simulink model "sphero_ver_01"  (R2020b)
settings: Solver=VariableStepAuto  StartTime=0.0  StopTime=10.0  RelTol=1e-3
libraries: pid_lib x1
settings Model: Creator=filip  LastModifiedBy=filip

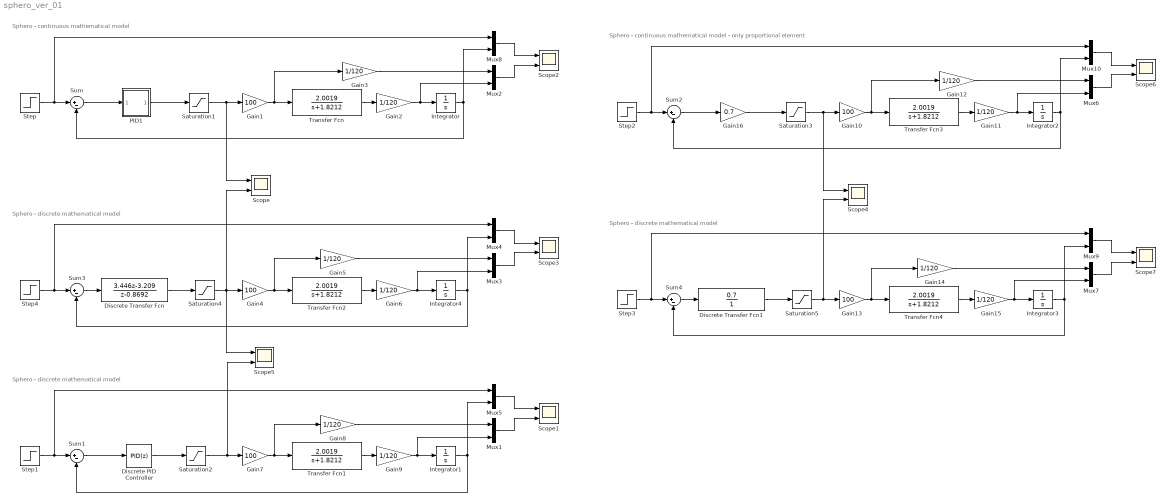
== system sphero_ver_01 ==
  note: Sphero - discrete mathematical model
  note: Sphero - continuous mathematical model
  note: Sphero - discrete mathematical model
  note: Sphero - continuous mathematical model - only proportional element
  note: Sphero - discrete mathematical model
  Discrete Transfer Fcn : DiscreteTransferFcn  Numerator=[3.446 -3.209]  Denominator=[1 -0.8692]  SampleTime=0.04
  Discrete Transfer Fcn1 : DiscreteTransferFcn  Numerator=[0.7]  Denominator=[1]  SampleTime=0.04
  Discrete PID Controller : pid_lib/PID Controller  Controller=PID  Form=Parallel  TimeDomain=Discrete-time  UseExternalTs=off  SampleTime=0.04  IntegratorMethod=Forward Euler  FilterMethod=Forward Euler  ControllerParametersSource=internal  P=1.81  I=0  D=0.5  UseFilter=on  N=3.5  TunerSelectOption=Transfer Function Based (PID Tuner App)  InitialConditionSource=internal  InitialConditionForIntegrator=0  InitialConditionForFilter=0  DifferentiatorICPrevScaledInput=0  ExternalReset=none  TrackingMode=off  Kt=1  LimitOutput=off  SatLimitsSource=internal  UpperSaturationLimit=inf  LowerSaturationLimit=-inf  LinearizeAsGain=off  AntiWindupMode=none  Kb=1  POutMin=[]  POutMax=[]  IOutMin=[]  IOutMax=[]  DOutMin=[]  DOutMax=[]  NOutMin=[]  NOutMax=[]  SumOutMin=[]  SumOutMax=[]  SaturationOutMin=[]  SaturationOutMax=[]  PParamMin=[]  PParamMax=[]  IParamMin=[]  IParamMax=[]  DParamMin=[]  DParamMax=[]  NParamMin=[]  NParamMax=[]  KbParamMin=[]  KbParamMax=[]  KtParamMin=[]  KtParamMax=[]  KbOutMin=[]  KbOutMax=[]  KtOutMin=[]  KtOutMax=[]  IntegratorOutMin=[]  IntegratorOutMax=[]  FilterOutMin=[]  FilterOutMax=[]  SumI1OutMin=[]  SumI1OutMax=[]  SumI2OutMin=[]  SumI2OutMax=[]  SumI3OutMin=[]  SumI3OutMax=[]  SumI4OutMin=[]  SumI4OutMax=[]  SumDOutMin=[]  SumDOutMax=[]  DifferentiatorOutMin=[]  DifferentiatorOutMax=[]  FilterDiffOutCoefMin=[]  FilterDiffOutCoefMax=[]  ReciprocalOutMin=[]  ReciprocalOutMax=[]  SumDenOutMin=[]  SumDenOutMax=[]  SumNumOutMin=[]  SumNumOutMax=[]  DivideOutMin=[]  DivideOutMax=[]  UdiffTsProdOutMin=[]  UdiffTsProdOutMax=[]  NTsProdOutMin=[]  NTsProdOutMax=[]  UintegralTsProdOutMin=[]  UintegralTsProdOutMax=[]  UngainTsProdOutMin=[]  UngainTsProdOutMax=[]  IntegratorContinuousStateAttributes=''  IntegratorStateMustResolveToSignalObject=off  IntegratorRTWStateStorageClass=Auto  FilterContinuousStateAttributes=''  FilterStateMustResolveToSignalObject=off  FilterRTWStateStorageClass=Auto  ParallelPVariant=InternalParameters  IdealPVariant=Disabled  IVariant=InternalParameters  DVariant=InternalParameters  IntegratorVariant=Discrete  SatVariant=Disabled  AWVariant=Passthrough  PCopyVariant=Disabled  TRVariant=Disabled  FdbkBlocksVariant=Forward  IdealPFdbkVariant=Disabled  SatFdbkVariant=Disabled  DerivativeFilterVariant=ForwardEulerFilter  NVariant=InternalParameters  NCopyVariant=Disabled  FilterICVariant=InternalICsFilter  IntegratorICVariant=InternalICs  ExternalResetVariant=Disabled  TRSumVariant=Passthrough  SumFdbkVariant=Disabled  SumVariant=Sum_PID  TsampFilterVariant=InternalTs  TsampNgainVariant=Passthrough  TsampIntegralVariant=Passthrough  ExternalSaturationOutDataTypeStr=Inherit: Same as second input
  Gain{1,4,7,10,13} (5 alike) : Gain  Gain=100
  Gain{2..3,5..6,8..9,11..12,14..15} (10 alike) : Gain  Gain=1/120
  Gain16 : Gain  Gain=0.7
  Integrator{,1..4} (5 alike) : Integrator
  Mux{1..10} (10 alike) : Mux  Inputs=2
  PID1 : Subsystem
  Saturation{1..5} (5 alike) : Saturate  UpperLimit=1  LowerLimit=-1
  Scope{,1..7} (8 alike) : Scope  NumInputPorts=2
  Step{,1..4} (5 alike) : Step  Time=0  SampleTime=0
  Sum{,1..4} (5 alike) : Sum  Inputs=|+-
  Transfer Fcn{,1..4} (5 alike) : TransferFcn  Numerator=[2.0019]  Denominator=[1 1.8212]
  wires:
  Transfer Fcn/1 -> Gain2/1
  Gain1/1 -> Gain3/1, Transfer Fcn/1
  Saturation4/1 -> Scope/2, Gain4/1, Scope5/1
  Discrete Transfer Fcn/1 -> Saturation4/1
  Transfer Fcn2/1 -> Gain6/1
  Sum3/1 -> Discrete Transfer Fcn/1
  Saturation1/1 -> Scope/1, Gain1/1
  Mux4/1 -> Scope3/1
  Mux2/1 -> Scope2/2
  Mux3/1 -> Scope3/2
  Step4/1 -> Mux4/1, Sum3/1
  Integrator4/1 -> Sum3/2, Mux4/2
  Gain4/1 -> Gain5/1, Transfer Fcn2/1
  Step/1 -> Mux8/1, Sum/1
  Integrator/1 -> Sum/2, Mux8/2
  Mux8/1 -> Scope2/1
  Gain2/1 -> Integrator/1, Mux2/2
  Gain3/1 -> Mux2/1
  Gain5/1 -> Mux3/1
  Gain6/1 -> Mux3/2, Integrator4/1
  Sum/1 -> PID1/1("  ")
  PID1/1(" ") -> Saturation1/1
  Transfer Fcn1/1 -> Gain9/1
  Step1/1 -> Mux5/1, Sum1/1
  Integrator1/1 -> Sum1/2, Mux5/2
  Gain9/1 -> Mux1/2, Integrator1/1
  Gain7/1 -> Gain8/1, Transfer Fcn1/1
  Gain8/1 -> Mux1/1
  Saturation2/1 -> Gain7/1, Scope5/2
  Mux1/1 -> Scope1/2
  Mux5/1 -> Scope1/1
  Sum1/1 -> Discrete PID Controller/1
  Discrete PID Controller/1 -> Saturation2/1
  Mux6/1 -> Scope6/2
  Mux10/1 -> Scope6/1
  Gain10/1 -> Gain12/1, Transfer Fcn3/1
  Gain11/1 -> Integrator2/1, Mux6/2
  Transfer Fcn4/1 -> Gain15/1
  Gain13/1 -> Gain14/1, Transfer Fcn4/1
  Sum4/1 -> Discrete Transfer Fcn1/1
  Gain12/1 -> Mux6/1
  Integrator2/1 -> Sum2/2, Mux10/2
  Step2/1 -> Mux10/1, Sum2/1
  Step3/1 -> Mux9/1, Sum4/1
  Discrete Transfer Fcn1/1 -> Saturation5/1
  Gain16/1 -> Saturation3/1
  Integrator3/1 -> Sum4/2, Mux9/2
  Saturation3/1 -> Scope4/1, Gain10/1
  Gain15/1 -> Mux7/2, Integrator3/1
  Saturation5/1 -> Scope4/2, Gain13/1
  Mux9/1 -> Scope7/1
  Sum2/1 -> Gain16/1
  Transfer Fcn3/1 -> Gain11/1
  Mux7/1 -> Scope7/2
  Gain14/1 -> Mux7/1

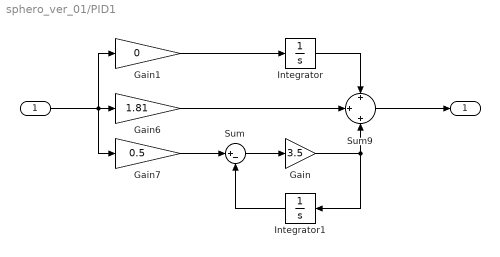
== system sphero_ver_01/PID1 ==
  "  " : Inport
  Gain : Gain  Gain=3.5
  Gain1 : Gain  Gain=0
  Gain6 : Gain  Gain=1.81
  Gain7 : Gain  Gain=0.5
  Integrator : Integrator
  Integrator1 : Integrator
  Sum : Sum  Inputs=|+-
  Sum9 : Sum  Inputs=+|+|+
  " " : Outport
  wires:
  Sum9/1 -> " "/1
  Gain6/1 -> Sum9/2
  "  "/1 -> Gain7/1, Gain1/1, Gain6/1
  Integrator/1 -> Sum9/1
  Gain1/1 -> Integrator/1
  Sum/1 -> Gain/1
  Gain7/1 -> Sum/1
  Gain/1 -> Integrator1/1, Sum9/3
  Integrator1/1 -> Sum/2
